simulink model "ExtDem_SelectParameter"  (R2016b)
settings: configuration reference "CodeGenConfigSet" (kept outside this file)
values from neighbouring files (symbols this model uses):
  ExtDem_facFdbk_CUR = Calibration.Parameter    [init_ExtDem_SelectParameter.m]
  ExtDem_facFdbk_CURX = Calibration.Parameter    [init_ExtDem_SelectParameter.m]
  ExtDem_facFdbkLimit_C = Calibration.Parameter    [init_ExtDem_SelectParameter.m]
  ExtDem_facFdbkParSet0_C = Calibration.Parameter    [init_ExtDem_SelectParameter.m]
  ExtDem_facFdbkParSet1_C = Calibration.Parameter    [init_ExtDem_SelectParameter.m]
  ExtDem_facFdbkParSet2_C = Calibration.Parameter    [init_ExtDem_SelectParameter.m]
  ExtDem_facFdbkParSet3_C = Calibration.Parameter    [init_ExtDem_SelectParameter.m]
  ExtDem_facFdbkParSet4_C = Calibration.Parameter    [init_ExtDem_SelectParameter.m]
  ExtDem_facFdbkParSet5_C = Calibration.Parameter    [init_ExtDem_SelectParameter.m]
  ExtDem_facFdbkParSet6_C = Calibration.Parameter    [init_ExtDem_SelectParameter.m]
  ExtDem_facFdbkParSet7_C = Calibration.Parameter    [init_ExtDem_SelectParameter.m]
  ExtDem_facNAvrgPT1CorFac_C = Calibration.Parameter    [init_ExtDem_SelectParameter.m]
  ExtDem_facTrqPT1CorFac_C = Calibration.Parameter    [init_ExtDem_SelectParameter.m]
  ExtDem_KiCorTempFac_MAP = Calibration.Parameter    [init_ExtDem_SelectParameter.m]
  ExtDem_KiCorTempFac_MAPX = Calibration.Parameter    [init_ExtDem_SelectParameter.m]
  ExtDem_KiCorTempFac_MAPY = Calibration.Parameter    [init_ExtDem_SelectParameter.m]
  ExtDem_KiCorTrqFac_MAP = Calibration.Parameter    [init_ExtDem_SelectParameter.m]
  ExtDem_KiCorTrqFac_MAPX = Calibration.Parameter    [init_ExtDem_SelectParameter.m]
  ExtDem_KiCorTrqFac_MAPY = Calibration.Parameter    [init_ExtDem_SelectParameter.m]
  ExtDem_KpCorTempFac_MAP = Calibration.Parameter    [init_ExtDem_SelectParameter.m]
  ExtDem_KpCorTempFac_MAPX = Calibration.Parameter    [init_ExtDem_SelectParameter.m]
  ExtDem_KpCorTempFac_MAPY = Calibration.Parameter    [init_ExtDem_SelectParameter.m]
  ExtDem_KpCorTrqFac_MAP = Calibration.Parameter    [init_ExtDem_SelectParameter.m]
  ExtDem_KpCorTrqFac_MAPX = Calibration.Parameter    [init_ExtDem_SelectParameter.m]
  ExtDem_KpCorTrqFac_MAPY = Calibration.Parameter    [init_ExtDem_SelectParameter.m]
  ExtDem_Par0Cfg_C = Calibration.Parameter    [init_ExtDem_SelectParameter.m]
  ExtDem_Par0dnAccLim_C = Calibration.Parameter    [init_ExtDem_SelectParameter.m]
  ExtDem_Par0dnDeclLim_C = Calibration.Parameter    [init_ExtDem_SelectParameter.m]
  ExtDem_Par0dnDeclLimBrk_C = Calibration.Parameter    [init_ExtDem_SelectParameter.m]
  ExtDem_Par0FacFdbkTrqLosHi_C = Calibration.Parameter    [init_ExtDem_SelectParameter.m]
  ExtDem_Par0FacFdbkTrqLosLo_C = Calibration.Parameter    [init_ExtDem_SelectParameter.m]
  ExtDem_Par0IKi_C = Calibration.Parameter    [init_ExtDem_SelectParameter.m]
  ExtDem_Par0IKiNeg_C = Calibration.Parameter    [init_ExtDem_SelectParameter.m]
  ExtDem_Par0IKiPos_C = Calibration.Parameter    [init_ExtDem_SelectParameter.m]
  ExtDem_Par0InrtVeh_C = Calibration.Parameter    [init_ExtDem_SelectParameter.m]
  ExtDem_Par0nIWinNeg_C = Calibration.Parameter    [init_ExtDem_SelectParameter.m]
  ExtDem_Par0nIWinPos_C = Calibration.Parameter    [init_ExtDem_SelectParameter.m]
  ExtDem_Par0nPWinNeg_C = Calibration.Parameter    [init_ExtDem_SelectParameter.m]
  ExtDem_Par0nPWinPos_C = Calibration.Parameter    [init_ExtDem_SelectParameter.m]
  ExtDem_Par0PKp_C = Calibration.Parameter    [init_ExtDem_SelectParameter.m]
  ExtDem_Par0PKpNeg_C = Calibration.Parameter    [init_ExtDem_SelectParameter.m]
  ExtDem_Par0PKpPos_C = Calibration.Parameter    [init_ExtDem_SelectParameter.m]
  ExtDem_Par0TiFltTrqLosEst_C = Calibration.Parameter    [init_ExtDem_SelectParameter.m]
  ExtDem_Par1Cfg_C = Calibration.Parameter    [init_ExtDem_SelectParameter.m]
  ExtDem_Par1dnAccLim_C = Calibration.Parameter    [init_ExtDem_SelectParameter.m]
  ExtDem_Par1dnDeclLim_C = Calibration.Parameter    [init_ExtDem_SelectParameter.m]
  ExtDem_Par1dnDeclLimBrk_C = Calibration.Parameter    [init_ExtDem_SelectParameter.m]
  ExtDem_Par1FacFdbkTrqLosHi_C = Calibration.Parameter    [init_ExtDem_SelectParameter.m]
  ExtDem_Par1FacFdbkTrqLosLo_C = Calibration.Parameter    [init_ExtDem_SelectParameter.m]
  ExtDem_Par1IKi_C = Calibration.Parameter    [init_ExtDem_SelectParameter.m]
  ExtDem_Par1IKiNeg_C = Calibration.Parameter    [init_ExtDem_SelectParameter.m]
  ExtDem_Par1IKiPos_C = Calibration.Parameter    [init_ExtDem_SelectParameter.m]
  ExtDem_Par1InrtVeh_C = Calibration.Parameter    [init_ExtDem_SelectParameter.m]
  ExtDem_Par1nIWinNeg_C = Calibration.Parameter    [init_ExtDem_SelectParameter.m]
  ExtDem_Par1nIWinPos_C = Calibration.Parameter    [init_ExtDem_SelectParameter.m]
  ExtDem_Par1nPWinNeg_C = Calibration.Parameter    [init_ExtDem_SelectParameter.m]
  ExtDem_Par1nPWinPos_C = Calibration.Parameter    [init_ExtDem_SelectParameter.m]
  ExtDem_Par1PKp_C = Calibration.Parameter    [init_ExtDem_SelectParameter.m]
  ExtDem_Par1PKpNeg_C = Calibration.Parameter    [init_ExtDem_SelectParameter.m]
  ExtDem_Par1PKpPos_C = Calibration.Parameter    [init_ExtDem_SelectParameter.m]
  ExtDem_Par1TiFltTrqLosEst_C = Calibration.Parameter    [init_ExtDem_SelectParameter.m]
  ExtDem_Par2Cfg_C = Calibration.Parameter    [init_ExtDem_SelectParameter.m]
  ExtDem_Par2dnAccLim_C = Calibration.Parameter    [init_ExtDem_SelectParameter.m]
  ExtDem_Par2dnDeclLim_C = Calibration.Parameter    [init_ExtDem_SelectParameter.m]
  ExtDem_Par2dnDeclLimBrk_C = Calibration.Parameter    [init_ExtDem_SelectParameter.m]
  ExtDem_Par2FacFdbkTrqLosHi_C = Calibration.Parameter    [init_ExtDem_SelectParameter.m]
  ExtDem_Par2FacFdbkTrqLosLo_C = Calibration.Parameter    [init_ExtDem_SelectParameter.m]
  ExtDem_Par2IKi_C = Calibration.Parameter    [init_ExtDem_SelectParameter.m]
  ExtDem_Par2IKiNeg_C = Calibration.Parameter    [init_ExtDem_SelectParameter.m]
  ExtDem_Par2IKiPos_C = Calibration.Parameter    [init_ExtDem_SelectParameter.m]
  ExtDem_Par2InrtVeh_C = Calibration.Parameter    [init_ExtDem_SelectParameter.m]
  ExtDem_Par2nIWinNeg_C = Calibration.Parameter    [init_ExtDem_SelectParameter.m]
  ExtDem_Par2nIWinPos_C = Calibration.Parameter    [init_ExtDem_SelectParameter.m]
  ExtDem_Par2nPWinNeg_C = Calibration.Parameter    [init_ExtDem_SelectParameter.m]
  ExtDem_Par2nPWinPos_C = Calibration.Parameter    [init_ExtDem_SelectParameter.m]
  ExtDem_Par2PKp_C = Calibration.Parameter    [init_ExtDem_SelectParameter.m]
  ExtDem_Par2PKpNeg_C = Calibration.Parameter    [init_ExtDem_SelectParameter.m]
  ExtDem_Par2PKpPos_C = Calibration.Parameter    [init_ExtDem_SelectParameter.m]
  ExtDem_Par2TiFltTrqLosEst_C = Calibration.Parameter    [init_ExtDem_SelectParameter.m]
  ExtDem_Par3Cfg_C = Calibration.Parameter    [init_ExtDem_SelectParameter.m]
  ExtDem_Par3dnAccLim_C = Calibration.Parameter    [init_ExtDem_SelectParameter.m]
  ExtDem_Par3dnDeclLim_C = Calibration.Parameter    [init_ExtDem_SelectParameter.m]
  ExtDem_Par3dnDeclLimBrk_C = Calibration.Parameter    [init_ExtDem_SelectParameter.m]
  ExtDem_Par3FacFdbkTrqLosHi_C = Calibration.Parameter    [init_ExtDem_SelectParameter.m]
  ExtDem_Par3FacFdbkTrqLosLo_C = Calibration.Parameter    [init_ExtDem_SelectParameter.m]
  ExtDem_Par3IKi_C = Calibration.Parameter    [init_ExtDem_SelectParameter.m]
  ExtDem_Par3IKiNeg_C = Calibration.Parameter    [init_ExtDem_SelectParameter.m]
  ExtDem_Par3IKiPos_C = Calibration.Parameter    [init_ExtDem_SelectParameter.m]
  ExtDem_Par3InrtVeh_C = Calibration.Parameter    [init_ExtDem_SelectParameter.m]
  ExtDem_Par3nIWinNeg_C = Calibration.Parameter    [init_ExtDem_SelectParameter.m]
  ExtDem_Par3nIWinPos_C = Calibration.Parameter    [init_ExtDem_SelectParameter.m]
  ExtDem_Par3nPWinNeg_C = Calibration.Parameter    [init_ExtDem_SelectParameter.m]
  ExtDem_Par3nPWinPos_C = Calibration.Parameter    [init_ExtDem_SelectParameter.m]
  ExtDem_Par3PKp_C = Calibration.Parameter    [init_ExtDem_SelectParameter.m]
  ExtDem_Par3PKpNeg_C = Calibration.Parameter    [init_ExtDem_SelectParameter.m]
  ExtDem_Par3PKpPos_C = Calibration.Parameter    [init_ExtDem_SelectParameter.m]
  ExtDem_Par3TiFltTrqLosEst_C = Calibration.Parameter    [init_ExtDem_SelectParameter.m]
  ExtDem_Par4Cfg_C = Calibration.Parameter    [init_ExtDem_SelectParameter.m]
  ExtDem_Par4dnAccLim_C = Calibration.Parameter    [init_ExtDem_SelectParameter.m]
  ExtDem_Par4dnDeclLim_C = Calibration.Parameter    [init_ExtDem_SelectParameter.m]
  ExtDem_Par4dnDeclLimBrk_C = Calibration.Parameter    [init_ExtDem_SelectParameter.m]
  ExtDem_Par4FacFdbkTrqLosHi_C = Calibration.Parameter    [init_ExtDem_SelectParameter.m]
  ExtDem_Par4FacFdbkTrqLosLo_C = Calibration.Parameter    [init_ExtDem_SelectParameter.m]
  ExtDem_Par4IKi_C = Calibration.Parameter    [init_ExtDem_SelectParameter.m]
  ExtDem_Par4IKiNeg_C = Calibration.Parameter    [init_ExtDem_SelectParameter.m]
  ExtDem_Par4IKiPos_C = Calibration.Parameter    [init_ExtDem_SelectParameter.m]
  ExtDem_Par4InrtVeh_C = Calibration.Parameter    [init_ExtDem_SelectParameter.m]
  ExtDem_Par4nIWinNeg_C = Calibration.Parameter    [init_ExtDem_SelectParameter.m]
  ExtDem_Par4nIWinPos_C = Calibration.Parameter    [init_ExtDem_SelectParameter.m]
  ExtDem_Par4nPWinNeg_C = Calibration.Parameter    [init_ExtDem_SelectParameter.m]
  ExtDem_Par4nPWinPos_C = Calibration.Parameter    [init_ExtDem_SelectParameter.m]
  ExtDem_Par4PKp_C = Calibration.Parameter    [init_ExtDem_SelectParameter.m]
  ExtDem_Par4PKpNeg_C = Calibration.Parameter    [init_ExtDem_SelectParameter.m]
  ExtDem_Par4PKpPos_C = Calibration.Parameter    [init_ExtDem_SelectParameter.m]
  ExtDem_Par4TiFltTrqLosEst_C = Calibration.Parameter    [init_ExtDem_SelectParameter.m]
  ExtDem_Par5Cfg_C = Calibration.Parameter    [init_ExtDem_SelectParameter.m]
  ExtDem_Par5dnAccLim_C = Calibration.Parameter    [init_ExtDem_SelectParameter.m]
  ExtDem_Par5dnDeclLim_C = Calibration.Parameter    [init_ExtDem_SelectParameter.m]
  ExtDem_Par5dnDeclLimBrk_C = Calibration.Parameter    [init_ExtDem_SelectParameter.m]
  ExtDem_Par5FacFdbkTrqLosHi_C = Calibration.Parameter    [init_ExtDem_SelectParameter.m]
  ... (+56 more)
libraries: CXLib x7
(part 1 of 2)
settings Model: Creator=dulinggang  LastModifiedBy=xuxingpei
settings ConfigSetRef: SourceLocation=Base Workspace

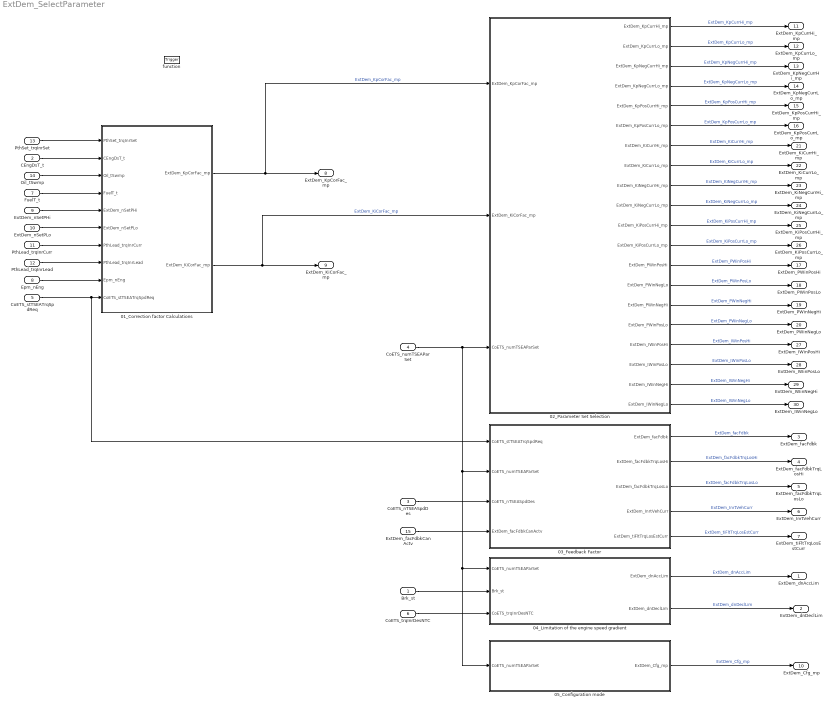
== system ExtDem_SelectParameter ==
  Brk_st : Inport  Description=Brake switch state  OutMin=0  OutMax=255  OutDataTypeStr=State_uint8
  CEngDsT_t : Inport  Tag=deg  Description=engine coolant temperature after filter  Port=2  OutMin=-200  OutMax=200  OutDataTypeStr=Temp_deg
  CoETS_nTSEASpdDes : Inport  Tag=rpm  Description=The desired/control engine speed requested from TSC1 CAN messages  Port=3  OutMin=0  OutMax=6000  OutDataTypeStr=EngSpeed_rpm
  CoETS_numTSEAParSet : Inport  Description=Number of requested parameter set for Engine speed governor  Port=4  OutMin=0  OutMax=255  OutDataTypeStr=State_uint8
  CoETS_stTSEATrqSpdReq : Inport  Description=Status of information about torque and speed intervention  Port=5  OutMin=0  OutMax=65535  OutDataTypeStr=State_uint16
  CoETS_trqInrDesNTC : Inport  Tag=Nm  Description=Additional desired engine friction Nm  Port=6  OutMin=-3276  OutMax=3276  OutDataTypeStr=Trq_Nm
  FuelT_t : Inport  Tag=deg  Description=EngPrt_PrtLimOvht:Temperature of fuel  Port=7  OutMin=-50  OutMax=150  OutDataTypeStr=Temp_deg
  Epm_nEng : Inport  Tag=rpm  Description=Engine speed  Port=8  OutMin=0  OutMax=6000  OutDataTypeStr=EngSpeed_rpm
  ExtDem_nSetPHi : Inport  Tag=rpm  Description=Higher limit of external demand set point speed  Port=9  OutMin=0  OutMax=6000  OutDataTypeStr=EngSpeed_rpm
  ExtDem_nSetPLo : Inport  Tag=rpm  Description=Lower limit of external demand set point speed  Port=10  OutMin=0  OutMax=6000  OutDataTypeStr=EngSpeed_rpm
  PthLead_trqInrCurr : Inport  Tag=Nm  Description=Actual percent engine torque  Port=11  OutMin=-3000  OutMax=3000  OutDataTypeStr=Trq_Nm
  PthLead_trqInrLead : Inport  Tag=Nm  Description=Inner torque lead value  Port=12  OutMin=-3000  OutMax=3000  OutDataTypeStr=Trq_Nm
  PthSet_trqInrSet : Inport  Tag=Nm  Description=Inner torque set value after monitoring limitation  Port=13  OutMin=-3000  OutMax=3276.7  OutDataTypeStr=Trq_Nm
  Oil_tSwmp : Inport  Tag=deg  Description=Oil temperature in oil sump  Port=14  OutMin=-50  OutMax=200  OutDataTypeStr=Temp_deg
  ExtDem_facFdbkCanActv : Inport  Tag=rpm/Nm  Description=External intervention feedback factor from CAN  Port=15  OutMin=-20  OutMax=20  OutDataTypeStr=FdbkNm2rpm_rpm_Nm
  function : TriggerPort  TriggerType=function-call  VariantControl=Variant
  "01_Correction factor Calculations " : Subsystem
  02_Parameter Set Selection : Subsystem
  "03_Feedback Factor " : Subsystem
  "04_Limitation of the engine speed gradient " : Subsystem
  "05_Conﬁguration mode " : Subsystem
  ExtDem_dnAccLim : Outport  Tag=rpm/s  Description=Maximum permissible acceleration (Engine speed)  OutMin=-12000  OutMax=12000  OutDataTypeStr=EngSpeed_rpm_s
  ExtDem_dnDeclLim : Outport  Tag=rpm/s  Description=Maximum permissible deceleration (Engine speed)  Port=2  OutMin=-12000  OutMax=12000  OutDataTypeStr=EngSpeed_rpm_s
  ExtDem_facFdbk : Outport  Tag=rpm/Nm  Description=External intervention feedback factor  Port=3  OutMin=-20  OutMax=20  OutDataTypeStr=FdbkNm2rpm_rpm_Nm
  ExtDem_facFdbkTrqLosHi : Outport  Tag=rpm/Nm  Description=inner feedback factor for the upper setpoint  Port=4  OutMin=-20  OutMax=20  OutDataTypeStr=FdbkNm2rpm_rpm_Nm
  ExtDem_facFdbkTrqLosLo : Outport  Tag=rpm/Nm  Description=inner feedback factor for the lower setpoint  Port=5  OutMin=-20  OutMax=20  OutDataTypeStr=FdbkNm2rpm_rpm_Nm
  ExtDem_InrtVehCurr : Outport  Tag=Nm/(rpm/s)  Description=Mass inirtia for EISGov torque loss estimation  Port=6  OutMin=-50  OutMax=50  OutDataTypeStr=HLSDem_Inrt
  ExtDem_tiFltTrqLosEstCurr : Outport  Tag=s  Description=Time constant for EISGov torque loss calculation  Port=7  OutMin=-180  OutMax=180  OutDataTypeStr=Time_s
  ExtDem_KpCorFac_mp : Outport  Description=Current small signal gain for the P component  Port=8  OutMin=-30  OutMax=30  OutDataTypeStr=Factor
  ExtDem_KiCorFac_mp : Outport  Description=Correction factor for I gain  Port=9  OutMin=-30  OutMax=30  OutDataTypeStr=Factor
  ExtDem_Cfg_mp : Outport  Description=Configuration for EISGov structure  Port=10  OutMin=0  OutMax=255  OutDataTypeStr=State_uint8
  ExtDem_KpCurrHi_mp : Outport  Tag=Nm/rpm  Description=Current small signal gain for the P higher component  Port=11  OutMin=-10000  OutMax=10000  OutDataTypeStr=HLSDem_Kp
  ExtDem_KpCurrLo_mp : Outport  Tag=Nm/rpm  Description=Current small signal gain for the P lower component  Port=12  OutMin=-10000  OutMax=10000  OutDataTypeStr=HLSDem_Kp
  ExtDem_KpNegCurrHi_mp : Outport  Tag=Nm/rpm  Description=Current negative large signal gain for the P higher component  Port=13  OutMin=-10000  OutMax=10000  OutDataTypeStr=HLSDem_Kp
  ExtDem_KpNegCurrLo_mp : Outport  Tag=Nm/rpm  Description=Current negative large signal gain for the lower P component  Port=14  OutMin=-10000  OutMax=10000  OutDataTypeStr=HLSDem_Kp
  ExtDem_KpPosCurrHi_mp : Outport  Tag=Nm/rpm  Description=Current positive large signal gain for the P higher component  Port=15  OutMin=-10000  OutMax=10000  OutDataTypeStr=HLSDem_Kp
  ExtDem_KpPosCurrLo_mp : Outport  Tag=Nm/rpm  Description=Current positive large signal gain for the P lower component  Port=16  OutMin=-10000  OutMax=10000  OutDataTypeStr=HLSDem_Kp
  ExtDem_PWinPosHi : Outport  Tag=rpm  Description=Positive small signal window for proportional higher component  Port=17  OutMin=-1000  OutMax=1000  OutDataTypeStr=EngSpeed_rpm
  ExtDem_PWinPosLo : Outport  Tag=rpm  Description=Positive small signal window for proportional lower component  Port=18  OutMin=-1000  OutMax=1000  OutDataTypeStr=EngSpeed_rpm
  ExtDem_PWinNegHi : Outport  Tag=rpm  Description=Negative small signal window for proportional higher component  Port=19  OutMin=-1000  OutMax=1000  OutDataTypeStr=EngSpeed_rpm
  ExtDem_PWinNegLo : Outport  Tag=rpm  Description=Negative small signal window for proportional lower component  Port=20  OutMin=-1000  OutMax=1000  OutDataTypeStr=EngSpeed_rpm
  ExtDem_KiCurrHi_mp : Outport  Tag=Nm/(rpm*s)  Description=Current small signal gain for the I higher component  Port=21  OutMin=-18000  OutMax=18000  OutDataTypeStr=HLSDem_Ki
  ExtDem_KiCurrLo_mp : Outport  Tag=Nm/(rpm*s)  Description=Current small signal gain for the I lower component  Port=22  OutMin=-18000  OutMax=18000  OutDataTypeStr=HLSDem_Ki
  ExtDem_KiNegCurrHi_mp : Outport  Tag=Nm/(rpm*s)  Description=Current negative large signal gain for the I higher component  Port=23  OutMin=-18000  OutMax=18000  OutDataTypeStr=HLSDem_Ki
  ExtDem_KiNegCurrLo_mp : Outport  Tag=Nm/(rpm*s)  Description=Current negative large signal gain for the I lower component  Port=24  OutMin=-18000  OutMax=18000  OutDataTypeStr=HLSDem_Ki
  ExtDem_KiPosCurrHi_mp : Outport  Tag=Nm/(rpm*s)  Description=Current positive large signal gain for the I higher component  Port=25  OutMin=-18000  OutMax=18000  OutDataTypeStr=HLSDem_Ki
  ExtDem_KiPosCurrLo_mp : Outport  Tag=Nm/(rpm*s)  Description=Current positive large signal gain for the I lower component  Port=26  OutMin=-18000  OutMax=18000  OutDataTypeStr=HLSDem_Ki
  ExtDem_IWinPosHi : Outport  Tag=rpm  Description=Positive small signal window for integral higher component  Port=27  OutMin=-1000  OutMax=1000  OutDataTypeStr=EngSpeed_rpm
  ExtDem_IWinPosLo : Outport  Tag=rpm  Description=Positive small signal window for integral lower component  Port=28  OutMin=-1000  OutMax=1000  OutDataTypeStr=EngSpeed_rpm
  ExtDem_IWinNegHi : Outport  Tag=rpm  Description=Negative small signal window for integral higher component  Port=29  OutMin=-1000  OutMax=1000  OutDataTypeStr=EngSpeed_rpm
  ExtDem_IWinNegLo : Outport  Tag=rpm  Description=Negative small signal window for integral lower component  Port=30  OutMin=-1000  OutMax=1000  OutDataTypeStr=EngSpeed_rpm
  wires:
  "03_Feedback Factor "/1(ExtDem_facFdbk) -> ExtDem_facFdbk/1  "ExtDem_facFdbk"
  "03_Feedback Factor "/2(ExtDem_facFdbkTrqLosHi) -> ExtDem_facFdbkTrqLosHi/1  "ExtDem_facFdbkTrqLosHi"
  "03_Feedback Factor "/3(ExtDem_facFdbkTrqLosLo) -> ExtDem_facFdbkTrqLosLo/1  "ExtDem_facFdbkTrqLosLo"
  "03_Feedback Factor "/4(ExtDem_InrtVehCurr) -> ExtDem_InrtVehCurr/1  "ExtDem_InrtVehCurr"
  "01_Correction factor Calculations "/1(ExtDem_KpCorFac_mp) -> ExtDem_KpCorFac_mp/1, 02_Parameter Set Selection/1(ExtDem_KpCorFac_mp)  "ExtDem_KpCorFac_mp"
  "01_Correction factor Calculations "/2(ExtDem_KiCorFac_mp) -> ExtDem_KiCorFac_mp/1, 02_Parameter Set Selection/2(ExtDem_KiCorFac_mp)  "ExtDem_KiCorFac_mp"
  "05_Conﬁguration mode "/1(ExtDem_Cfg_mp) -> ExtDem_Cfg_mp/1  "ExtDem_Cfg_mp"
  CoETS_stTSEATrqSpdReq/1 -> "03_Feedback Factor "/1(CoETS_stTSEATrqSpdReq), "01_Correction factor Calculations "/10(CoETS_stTSEATrqSpdReq)
  ExtDem_nSetPHi/1 -> "01_Correction factor Calculations "/5(ExtDem_nSetPHi)
  PthLead_trqInrCurr/1 -> "01_Correction factor Calculations "/7(PthLead_trqInrCurr)
  PthLead_trqInrLead/1 -> "01_Correction factor Calculations "/8(PthLead_trqInrLead)
  PthSet_trqInrSet/1 -> "01_Correction factor Calculations "/1(PthSet_trqInrSet)
  CEngDsT_t/1 -> "01_Correction factor Calculations "/2(CEngDsT_t)
  Oil_tSwmp/1 -> "01_Correction factor Calculations "/3(Oil_tSwmp)
  FuelT_t/1 -> "01_Correction factor Calculations "/4(FuelT_t)
  CoETS_numTSEAParSet/1 -> "03_Feedback Factor "/2(CoETS_numTSEAParSet), "05_Conﬁguration mode "/1(CoETS_numTSEAParSet), "04_Limitation of the engine speed gradient "/1(CoETS_numTSEAParSet), 02_Parameter Set Selection/3(CoETS_numTSEAParSet)
  CoETS_nTSEASpdDes/1 -> "03_Feedback Factor "/3(CoETS_nTSEASpdDes)
  Brk_st/1 -> "04_Limitation of the engine speed gradient "/2(Brk_st)
  CoETS_trqInrDesNTC/1 -> "04_Limitation of the engine speed gradient "/3(CoETS_trqInrDesNTC)
  "04_Limitation of the engine speed gradient "/1(ExtDem_dnAccLim) -> ExtDem_dnAccLim/1  "ExtDem_dnAccLim"
  "04_Limitation of the engine speed gradient "/2(ExtDem_dnDeclLim) -> ExtDem_dnDeclLim/1  "ExtDem_dnDeclLim"
  Epm_nEng/1 -> "01_Correction factor Calculations "/9(Epm_nEng)
  ExtDem_nSetPLo/1 -> "01_Correction factor Calculations "/6(ExtDem_nSetPLo)
  02_Parameter Set Selection/1(ExtDem_KpCurrHi_mp) -> ExtDem_KpCurrHi_mp/1  "ExtDem_KpCurrHi_mp"
  02_Parameter Set Selection/2(ExtDem_KpCurrLo_mp) -> ExtDem_KpCurrLo_mp/1  "ExtDem_KpCurrLo_mp"
  02_Parameter Set Selection/3(ExtDem_KpNegCurrHi_mp) -> ExtDem_KpNegCurrHi_mp/1  "ExtDem_KpNegCurrHi_mp"
  02_Parameter Set Selection/4(ExtDem_KpNegCurrLo_mp) -> ExtDem_KpNegCurrLo_mp/1  "ExtDem_KpNegCurrLo_mp"
  02_Parameter Set Selection/5(ExtDem_KpPosCurrHi_mp) -> ExtDem_KpPosCurrHi_mp/1  "ExtDem_KpPosCurrHi_mp"
  02_Parameter Set Selection/6(ExtDem_KpPosCurrLo_mp) -> ExtDem_KpPosCurrLo_mp/1  "ExtDem_KpPosCurrLo_mp"
  02_Parameter Set Selection/7(ExtDem_KiCurrHi_mp) -> ExtDem_KiCurrHi_mp/1  "ExtDem_KiCurrHi_mp"
  02_Parameter Set Selection/8(ExtDem_KiCurrLo_mp) -> ExtDem_KiCurrLo_mp/1  "ExtDem_KiCurrLo_mp"
  02_Parameter Set Selection/9(ExtDem_KiNegCurrHi_mp) -> ExtDem_KiNegCurrHi_mp/1  "ExtDem_KiNegCurrHi_mp"
  02_Parameter Set Selection/10(ExtDem_KiNegCurrLo_mp) -> ExtDem_KiNegCurrLo_mp/1  "ExtDem_KiNegCurrLo_mp"
  02_Parameter Set Selection/11(ExtDem_KiPosCurrHi_mp) -> ExtDem_KiPosCurrHi_mp/1  "ExtDem_KiPosCurrHi_mp"
  02_Parameter Set Selection/12(ExtDem_KiPosCurrLo_mp) -> ExtDem_KiPosCurrLo_mp/1  "ExtDem_KiPosCurrLo_mp"
  ExtDem_facFdbkCanActv/1 -> "03_Feedback Factor "/4(ExtDem_facFdbkCanActv)
  "03_Feedback Factor "/5(ExtDem_tiFltTrqLosEstCurr) -> ExtDem_tiFltTrqLosEstCurr/1  "ExtDem_tiFltTrqLosEstCurr"
  02_Parameter Set Selection/17(ExtDem_IWinPosHi) -> ExtDem_IWinPosHi/1  "ExtDem_IWinPosHi"
  02_Parameter Set Selection/18(ExtDem_IWinPosLo) -> ExtDem_IWinPosLo/1  "ExtDem_IWinPosLo"
  02_Parameter Set Selection/19(ExtDem_IWinNegHi) -> ExtDem_IWinNegHi/1  "ExtDem_IWinNegHi"
  02_Parameter Set Selection/20(ExtDem_IWinNegLo) -> ExtDem_IWinNegLo/1  "ExtDem_IWinNegLo"
  02_Parameter Set Selection/13(ExtDem_PWinPosHi) -> ExtDem_PWinPosHi/1  "ExtDem_PWinPosHi"
  02_Parameter Set Selection/15(ExtDem_PWinNegHi) -> ExtDem_PWinNegHi/1  "ExtDem_PWinNegHi"
  02_Parameter Set Selection/14(ExtDem_PWinNegLo) -> ExtDem_PWinPosLo/1  "ExtDem_PWinPosLo"
  02_Parameter Set Selection/16(ExtDem_PWinPosLo) -> ExtDem_PWinNegLo/1  "ExtDem_PWinNegLo"

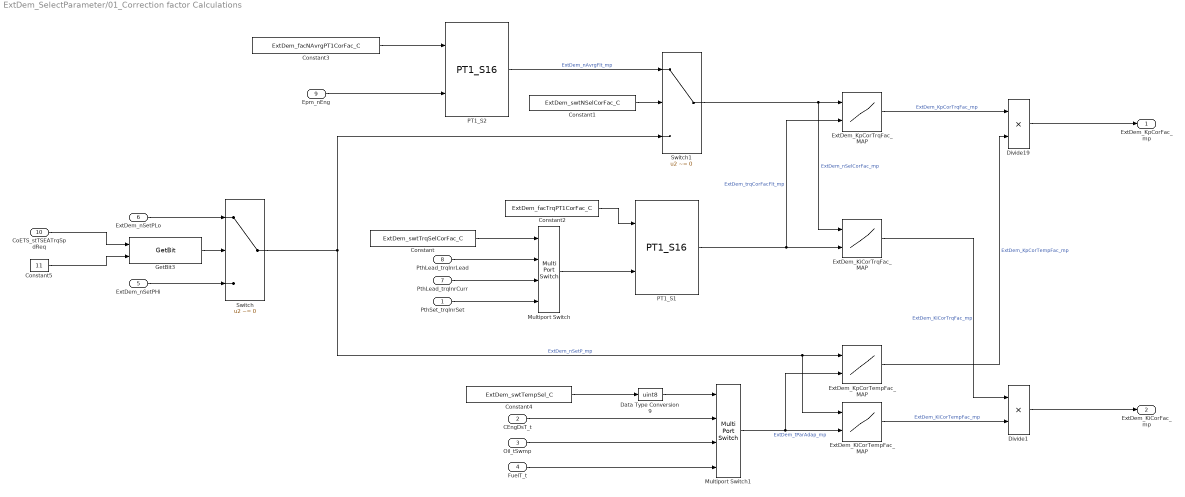
== system ExtDem_SelectParameter/01_Correction factor Calculations  ==
  PthSet_trqInrSet : Inport  Tag=Nm  Description=Inner torque set value after monitoring limitation  OutMin=-3000  OutMax=3276.7  OutDataTypeStr=Trq_Nm
  CEngDsT_t : Inport  Tag=deg  Description=engine coolant temperature after filter  Port=2  OutMin=-200  OutMax=200  OutDataTypeStr=Temp_deg
  Oil_tSwmp : Inport  Tag=deg  Description=Oil temperature in oil sump  Port=3  OutMin=-50  OutMax=200  OutDataTypeStr=Temp_deg
  FuelT_t : Inport  Tag=deg  Description=Engine temperature field  Port=4  OutMin=-3000  OutMax=3000  OutDataTypeStr=Temp_deg
  ExtDem_nSetPHi : Inport  Tag=rpm  Description=Higher limit of external demand set point speed  Port=5  OutMin=0  OutMax=6000  OutDataTypeStr=EngSpeed_rpm
  ExtDem_nSetPLo : Inport  Tag=rpm  Description=Lower limit of external demand set point speed  Port=6  OutMin=0  OutMax=6000  OutDataTypeStr=EngSpeed_rpm
  PthLead_trqInrCurr : Inport  Tag=Nm  Description=Actual percent engine torque  Port=7  OutMin=-3000  OutMax=3000  OutDataTypeStr=Trq_Nm
  PthLead_trqInrLead : Inport  Tag=Nm  Description=Inner torque lead value  Port=8  OutMin=-3000  OutMax=3000  OutDataTypeStr=Trq_Nm
  Epm_nEng : Inport  Tag=rpm  Description=Engine speed  Port=9  OutMin=0  OutMax=6000  OutDataTypeStr=EngSpeed_rpm
  CoETS_stTSEATrqSpdReq : Inport  Description=Status of information about torque and speed intervention  Port=10  OutMin=0  OutMax=65535  OutDataTypeStr=State_uint16
  Constant : Constant  Value=ExtDem_swtTrqSelCorFac_C
  Constant1 : Constant  Value=ExtDem_swtNSelCorFac_C
  Constant2 : Constant  Value=ExtDem_facTrqPT1CorFac_C
  Constant3 : Constant  Value=ExtDem_facNAvrgPT1CorFac_C
  Constant4 : Constant  Value=ExtDem_swtTempSel_C
  Constant5 : Constant  Value=11  OutDataTypeStr=Inherit: Inherit via back propagation
  Data Type Conversion9 : DataTypeConversion  OutDataTypeStr=uint8
  Divide1 : Product  Inputs=**  OutDataTypeStr=Factor  SaturateOnIntegerOverflow=on
  Divide19 : Product  Inputs=**  OutDataTypeStr=Factor  SaturateOnIntegerOverflow=on
  ExtDem_KiCorTempFac_MAP : Lookup_n-D  BreakpointsForDimension1=ExtDem_KiCorTempFac_MAPX  BreakpointsForDimension2=ExtDem_KiCorTempFac_MAPY  BeginIndexSearchUsingPreviousIndexResult=on  Table=ExtDem_KiCorTempFac_MAP  ExtrapMethod=Clip  UseLastTableValue=on  InternalRulePriority=Speed  OutDataTypeStr=Inherit: Inherit via back propagation  RndMeth=Simplest  SaturateOnIntegerOverflow=on
  ExtDem_KiCorTrqFac_MAP : Lookup_n-D  BreakpointsForDimension1=ExtDem_KiCorTrqFac_MAPX  BreakpointsForDimension2=ExtDem_KiCorTrqFac_MAPY  BeginIndexSearchUsingPreviousIndexResult=on  Table=ExtDem_KiCorTrqFac_MAP  ExtrapMethod=Clip  UseLastTableValue=on  InternalRulePriority=Speed  OutDataTypeStr=Inherit: Inherit via back propagation  RndMeth=Simplest  SaturateOnIntegerOverflow=on
  ExtDem_KpCorTempFac_MAP : Lookup_n-D  BreakpointsForDimension1=ExtDem_KpCorTempFac_MAPX  BreakpointsForDimension2=ExtDem_KpCorTempFac_MAPY  BeginIndexSearchUsingPreviousIndexResult=on  Table=ExtDem_KpCorTempFac_MAP  ExtrapMethod=Clip  UseLastTableValue=on  InternalRulePriority=Speed  OutDataTypeStr=Inherit: Inherit via back propagation  RndMeth=Simplest  SaturateOnIntegerOverflow=on
  ExtDem_KpCorTrqFac_MAP : Lookup_n-D  BreakpointsForDimension1=ExtDem_KpCorTrqFac_MAPX  BreakpointsForDimension2=ExtDem_KpCorTrqFac_MAPY  BeginIndexSearchUsingPreviousIndexResult=on  Table=ExtDem_KpCorTrqFac_MAP  ExtrapMethod=Clip  UseLastTableValue=on  InternalRulePriority=Speed  OutDataTypeStr=Inherit: Inherit via back propagation  RndMeth=Simplest  SaturateOnIntegerOverflow=on
  GetBit3 : CXLib/GetBit  dataTypeString=uint16  dataLength=0
      settings: AttributesFormatString=Get bit from %<dataTypeString>
  Multiport Switch : MultiPortSwitch  DataPortOrder=Zero-based contiguous
  Multiport Switch1 : MultiPortSwitch  DataPortOrder=Zero-based contiguous
  PT1_S1 : CXLib/PT1_S16
  PT1_S2 : CXLib/PT1_S16
  Switch : Switch  Criteria=u2 ~= 0
  Switch1 : Switch  Criteria=u2 ~= 0
  ExtDem_KpCorFac_mp : Outport  Description=Current small signal gain for the P component  OutMin=-30  OutMax=30  OutDataTypeStr=Factor
  ExtDem_KiCorFac_mp : Outport  Description=Correction factor for I gain  Port=2  OutMin=-30  OutMax=30  OutDataTypeStr=Factor
  wires:
  ExtDem_nSetPLo/1 -> Switch/1
  ExtDem_nSetPHi/1 -> Switch/3
  GetBit3/1 -> Switch/2
  Switch/1 -> Switch1/3, ExtDem_KiCorTempFac_MAP/1, ExtDem_KpCorTempFac_MAP/1  "ExtDem_nSetP_mp"
  PthSet_trqInrSet/1 -> Multiport Switch/4
  PthLead_trqInrCurr/1 -> Multiport Switch/3
  PthLead_trqInrLead/1 -> Multiport Switch/2
  Constant/1 -> Multiport Switch/1
  Multiport Switch/1 -> PT1_S1/2
  Epm_nEng/1 -> PT1_S2/2
  PT1_S2/1 -> Switch1/1  "ExtDem_nAvrgFlt_mp"
  Switch1/1 -> ExtDem_KiCorTrqFac_MAP/1, ExtDem_KpCorTrqFac_MAP/1  "ExtDem_nSelCorFac_mp"
  Constant1/1 -> Switch1/2
  Constant2/1 -> PT1_S1/1
  Constant3/1 -> PT1_S2/1
  ExtDem_KpCorTrqFac_MAP/1 -> Divide19/1  "ExtDem_KpCorTrqFac_mp"
  ExtDem_KiCorTrqFac_MAP/1 -> Divide1/1  "ExtDem_KiCorTrqFac_mp"
  CEngDsT_t/1 -> Multiport Switch1/2
  Oil_tSwmp/1 -> Multiport Switch1/3
  FuelT_t/1 -> Multiport Switch1/4
  Data Type Conversion9/1 -> Multiport Switch1/1
  Constant4/1 -> Data Type Conversion9/1
  Multiport Switch1/1 -> ExtDem_KiCorTempFac_MAP/2, ExtDem_KpCorTempFac_MAP/2  "ExtDem_tParAdap_mp"
  ExtDem_KpCorTempFac_MAP/1 -> Divide19/2  "ExtDem_KpCorTempFac_mp"
  ExtDem_KiCorTempFac_MAP/1 -> Divide1/2  "ExtDem_KiCorTempFac_mp"
  Divide19/1 -> ExtDem_KpCorFac_mp/1
  Divide1/1 -> ExtDem_KiCorFac_mp/1
  PT1_S1/1 -> ExtDem_KpCorTrqFac_MAP/2, ExtDem_KiCorTrqFac_MAP/2  "ExtDem_trqCorFacFlt_mp"
  Constant5/1 -> GetBit3/2
  CoETS_stTSEATrqSpdReq/1 -> GetBit3/1

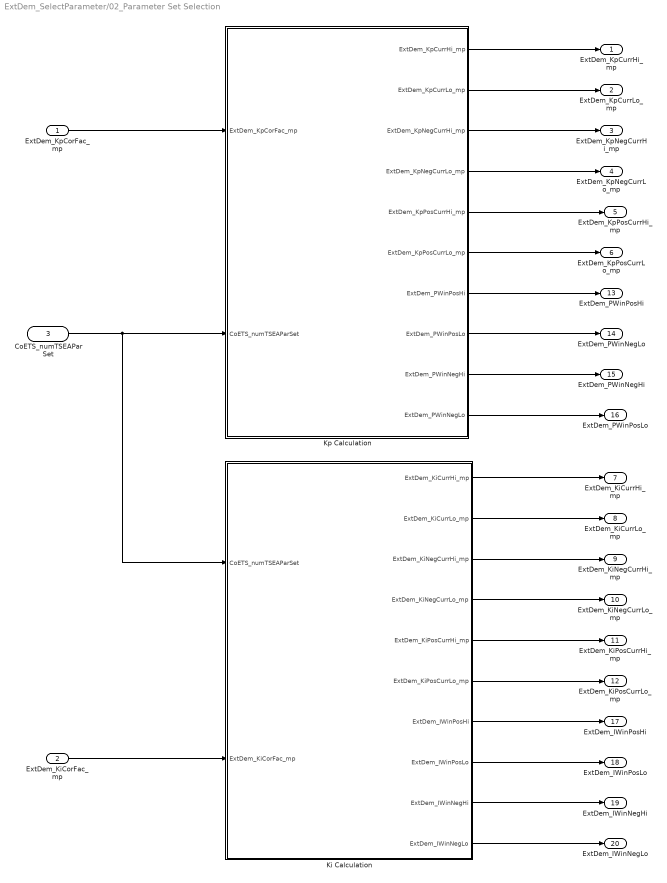
== system ExtDem_SelectParameter/02_Parameter Set Selection ==
  ExtDem_KpCorFac_mp : Inport  Description=Number of requested parameter set for Engine speed governor  OutMin=-30  OutMax=30  OutDataTypeStr=Factor
  ExtDem_KiCorFac_mp : Inport  Description=Number of requested parameter set for Engine speed governor  Port=2  OutMin=-30  OutMax=30  OutDataTypeStr=Factor
  CoETS_numTSEAParSet : Inport  Description=Number of requested parameter set for Engine speed governor  Port=3  OutMin=0  OutMax=255  OutDataTypeStr=uint8
  Ki Calculation : Subsystem
  "Kp Calculation " : Subsystem
  ExtDem_KpCurrHi_mp : Outport  Tag=Nm/rpm  Description=Current small signal gain for the P higher component  OutMin=-10000  OutMax=10000  OutDataTypeStr=HLSDem_Kp
  ExtDem_KpCurrLo_mp : Outport  Tag=Nm/rpm  Description=Current small signal gain for the P lower component  Port=2  OutMin=-10000  OutMax=10000  OutDataTypeStr=HLSDem_Kp
  ExtDem_KpNegCurrHi_mp : Outport  Tag=Nm/rpm  Description=Current negative large signal gain for the P higher component  Port=3  OutMin=-10000  OutMax=10000  OutDataTypeStr=HLSDem_Kp
  ExtDem_KpNegCurrLo_mp : Outport  Tag=Nm/rpm  Description=Current negative large signal gain for the lower P component  Port=4  OutMin=-10000  OutMax=10000  OutDataTypeStr=HLSDem_Kp
  ExtDem_KpPosCurrHi_mp : Outport  Tag=Nm/rpm  Description=Current positive large signal gain for the P higher component  Port=5  OutMin=-10000  OutMax=10000  OutDataTypeStr=HLSDem_Kp
  ExtDem_KpPosCurrLo_mp : Outport  Tag=Nm/rpm  Description=Current positive large signal gain for the P lower component  Port=6  OutMin=-10000  OutMax=10000  OutDataTypeStr=HLSDem_Kp
  ExtDem_KiCurrHi_mp : Outport  Tag=Nm/(rpm*s)  Description=Current small signal gain for the I higher component  Port=7  OutMin=-18000  OutMax=18000  OutDataTypeStr=HLSDem_Ki
  ExtDem_KiCurrLo_mp : Outport  Tag=Nm/(rpm*s)  Description=Current small signal gain for the I lower component  Port=8  OutMin=-18000  OutMax=18000  OutDataTypeStr=HLSDem_Ki
  ExtDem_KiNegCurrHi_mp : Outport  Tag=Nm/(rpm*s)  Description=Current negative large signal gain for the I higher component  Port=9  OutMin=-18000  OutMax=18000  OutDataTypeStr=HLSDem_Ki
  ExtDem_KiNegCurrLo_mp : Outport  Tag=Nm/(rpm*s)  Description=Current negative large signal gain for the I lower component  Port=10  OutMin=-18000  OutMax=18000  OutDataTypeStr=HLSDem_Ki
  ExtDem_KiPosCurrHi_mp : Outport  Tag=Nm/(rpm*s)  Description=Current positive large signal gain for the I higher component  Port=11  OutMin=-18000  OutMax=18000  OutDataTypeStr=HLSDem_Ki
  ExtDem_KiPosCurrLo_mp : Outport  Tag=Nm/(rpm*s)  Description=Current positive large signal gain for the I lower component  Port=12  OutMin=-18000  OutMax=18000  OutDataTypeStr=HLSDem_Ki
  ExtDem_PWinPosHi : Outport  Tag=rpm  Description=Positive small signal window for proportional higher component  Port=13  OutMin=-1000  OutMax=1000  OutDataTypeStr=EngSpeed_rpm
  ExtDem_PWinNegLo : Outport  Tag=rpm  Description=Negative small signal window for proportional lower component  Port=14  OutMin=-1000  OutMax=1000  OutDataTypeStr=EngSpeed_rpm
  ExtDem_PWinNegHi : Outport  Tag=rpm  Description=Negative small signal window for proportional higher component  Port=15  OutMin=-1000  OutMax=1000  OutDataTypeStr=EngSpeed_rpm
  ExtDem_PWinPosLo : Outport  Tag=rpm  Description=Positive small signal window for proportional lower component  Port=16  OutMin=-1000  OutMax=1000  OutDataTypeStr=EngSpeed_rpm
  ExtDem_IWinPosHi : Outport  Tag=rpm  Description=Positive small signal window for integral higher component  Port=17  OutMin=-1000  OutMax=1000  OutDataTypeStr=EngSpeed_rpm
  ExtDem_IWinPosLo : Outport  Tag=rpm  Description=Positive small signal window for integral lower component  Port=18  OutMin=-1000  OutMax=1000  OutDataTypeStr=EngSpeed_rpm
  ExtDem_IWinNegHi : Outport  Tag=rpm  Description=Negative small signal window for integral higher component  Port=19  OutMin=-1000  OutMax=1000  OutDataTypeStr=EngSpeed_rpm
  ExtDem_IWinNegLo : Outport  Tag=rpm  Description=Negative small signal window for integral lower component  Port=20  OutMin=-1000  OutMax=1000  OutDataTypeStr=EngSpeed_rpm
  wires:
  CoETS_numTSEAParSet/1 -> Ki Calculation/1(CoETS_numTSEAParSet), "Kp Calculation "/2(CoETS_numTSEAParSet)
  "Kp Calculation "/1(ExtDem_KpCurrHi_mp) -> ExtDem_KpCurrHi_mp/1
  "Kp Calculation "/2(ExtDem_KpCurrLo_mp) -> ExtDem_KpCurrLo_mp/1
  "Kp Calculation "/3(ExtDem_KpNegCurrHi_mp) -> ExtDem_KpNegCurrHi_mp/1
  "Kp Calculation "/4(ExtDem_KpNegCurrLo_mp) -> ExtDem_KpNegCurrLo_mp/1
  "Kp Calculation "/5(ExtDem_KpPosCurrHi_mp) -> ExtDem_KpPosCurrHi_mp/1
  "Kp Calculation "/6(ExtDem_KpPosCurrLo_mp) -> ExtDem_KpPosCurrLo_mp/1
  Ki Calculation/1(ExtDem_KiCurrHi_mp) -> ExtDem_KiCurrHi_mp/1
  Ki Calculation/2(ExtDem_KiCurrLo_mp) -> ExtDem_KiCurrLo_mp/1
  Ki Calculation/3(ExtDem_KiNegCurrHi_mp) -> ExtDem_KiNegCurrHi_mp/1
  Ki Calculation/4(ExtDem_KiNegCurrLo_mp) -> ExtDem_KiNegCurrLo_mp/1
  Ki Calculation/5(ExtDem_KiPosCurrHi_mp) -> ExtDem_KiPosCurrHi_mp/1
  Ki Calculation/6(ExtDem_KiPosCurrLo_mp) -> ExtDem_KiPosCurrLo_mp/1
  ExtDem_KpCorFac_mp/1 -> "Kp Calculation "/1(ExtDem_KpCorFac_mp)
  ExtDem_KiCorFac_mp/1 -> Ki Calculation/2(ExtDem_KiCorFac_mp)
  "Kp Calculation "/7(ExtDem_PWinPosHi) -> ExtDem_PWinPosHi/1
  "Kp Calculation "/9(ExtDem_PWinNegHi) -> ExtDem_PWinNegHi/1
  Ki Calculation/7(ExtDem_IWinPosHi) -> ExtDem_IWinPosHi/1
  Ki Calculation/8(ExtDem_IWinPosLo) -> ExtDem_IWinPosLo/1
  Ki Calculation/9(ExtDem_IWinNegHi) -> ExtDem_IWinNegHi/1
  Ki Calculation/10(ExtDem_IWinNegLo) -> ExtDem_IWinNegLo/1
  "Kp Calculation "/10(ExtDem_PWinNegLo) -> ExtDem_PWinPosLo/1
  "Kp Calculation "/8(ExtDem_PWinPosLo) -> ExtDem_PWinNegLo/1

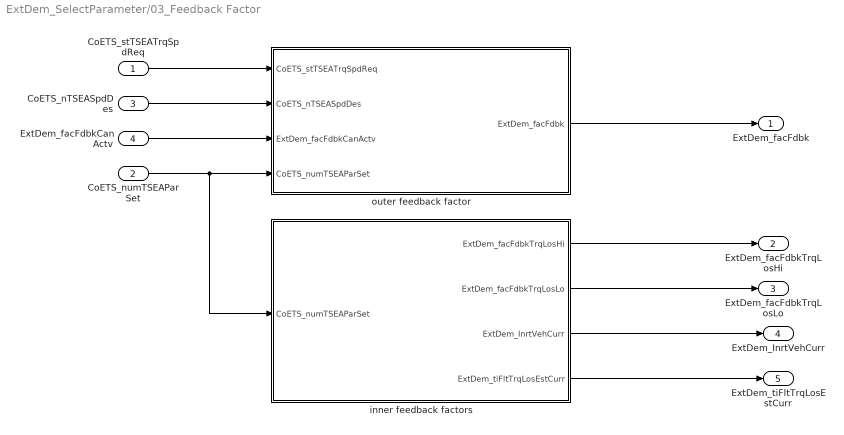
== system ExtDem_SelectParameter/03_Feedback Factor  ==
  CoETS_stTSEATrqSpdReq : Inport  Description=Status of information about torque and speed intervention  OutMin=0  OutMax=65535  OutDataTypeStr=State_uint16
  CoETS_numTSEAParSet : Inport  Description=Number of requested parameter set for Engine speed governor  Port=2  OutMin=0  OutMax=255  OutDataTypeStr=State_uint8
  CoETS_nTSEASpdDes : Inport  Tag=rpm  Description=The desired/control engine speed requested from TSC1 CAN messages  Port=3  OutMin=0  OutMax=6000  OutDataTypeStr=EngSpeed_rpm
  ExtDem_facFdbkCanActv : Inport  Tag=rpm/Nm  Description=External intervention feedback factor from CAN  Port=4  OutMin=-20  OutMax=20  OutDataTypeStr=FdbkNm2rpm_rpm_Nm
  " inner feedback factors " : Subsystem
  "outer feedback factor " : Subsystem
  ExtDem_facFdbk : Outport  Tag=rpm/Nm  Description=External intervention feedback factor  OutMin=-20  OutMax=20  OutDataTypeStr=FdbkNm2rpm_rpm_Nm
  ExtDem_facFdbkTrqLosHi : Outport  Tag=rpm/Nm  Description=inner feedback factor for the upper setpoint  Port=2  OutMin=-20  OutMax=20  OutDataTypeStr=FdbkNm2rpm_rpm_Nm
  ExtDem_facFdbkTrqLosLo : Outport  Tag=rpm/Nm  Description=inner feedback factor for the lower setpoint  Port=3  OutMin=-20  OutMax=20  OutDataTypeStr=FdbkNm2rpm_rpm_Nm
  ExtDem_InrtVehCurr : Outport  Tag=Nm/(rpm/s)  Description=Mass inirtia for EISGov torque loss estimation  Port=4  OutMin=-50  OutMax=50  OutDataTypeStr=HLSDem_Inrt
  ExtDem_tiFltTrqLosEstCurr : Outport  Tag=s  Description=Time constant for EISGov torque loss calculation  Port=5  OutMin=-180  OutMax=180  OutDataTypeStr=Time_s
  wires:
  CoETS_stTSEATrqSpdReq/1 -> "outer feedback factor "/1(CoETS_stTSEATrqSpdReq)
  CoETS_nTSEASpdDes/1 -> "outer feedback factor "/2(CoETS_nTSEASpdDes)
  "outer feedback factor "/1(ExtDem_facFdbk) -> ExtDem_facFdbk/1
  " inner feedback factors "/1(ExtDem_facFdbkTrqLosHi) -> ExtDem_facFdbkTrqLosHi/1
  " inner feedback factors "/2(ExtDem_facFdbkTrqLosLo) -> ExtDem_facFdbkTrqLosLo/1
  CoETS_numTSEAParSet/1 -> " inner feedback factors "/1(CoETS_numTSEAParSet), "outer feedback factor "/4(CoETS_numTSEAParSet)
  " inner feedback factors "/3(ExtDem_InrtVehCurr) -> ExtDem_InrtVehCurr/1
  ExtDem_facFdbkCanActv/1 -> "outer feedback factor "/3(ExtDem_facFdbkCanActv)
  " inner feedback factors "/4(ExtDem_tiFltTrqLosEstCurr) -> ExtDem_tiFltTrqLosEstCurr/1

== system ExtDem_SelectParameter/04_Limitation of the engine speed gradient  ==
  CoETS_numTSEAParSet : Inport  Description=Number of requested parameter set for Engine speed governor  OutMin=0  OutMax=255  OutDataTypeStr=State_uint8
  Brk_st : Inport  Description=Brake switch state  Port=2  OutMin=0  OutMax=255  OutDataTypeStr=State_uint8
  CoETS_trqInrDesNTC : Inport  Tag=Nm  Description=Additional desired engine friction Nm  Port=3  OutMin=-3276  OutMax=3276  OutDataTypeStr=Trq_Nm
  dnAccLim : Subsystem
  dnDecLim : Subsystem
  ExtDem_dnAccLim : Outport  Tag=rpm/s  Description=Maximum permissible acceleration (Engine speed)  OutMin=-12000  OutMax=12000  OutDataTypeStr=EngSpeed_rpm_s
  ExtDem_dnDeclLim : Outport  Tag=rpm/s  Description=Maximum permissible deceleration (Engine speed)  Port=2  OutMin=-12000  OutMax=12000  OutDataTypeStr=EngSpeed_rpm_s
  wires:
  CoETS_numTSEAParSet/1 -> dnDecLim/1(CoETS_numTSEAParSet), dnAccLim/1(CoETS_numTSEAParSet)
  dnAccLim/1(ExtDem_dnAccLim) -> ExtDem_dnAccLim/1
  dnDecLim/1(ExtDem_dnDeclLim) -> ExtDem_dnDeclLim/1
  Brk_st/1 -> dnDecLim/2(Brk_st)
  CoETS_trqInrDesNTC/1 -> dnDecLim/3(CoETS_trqInrDesNTC)

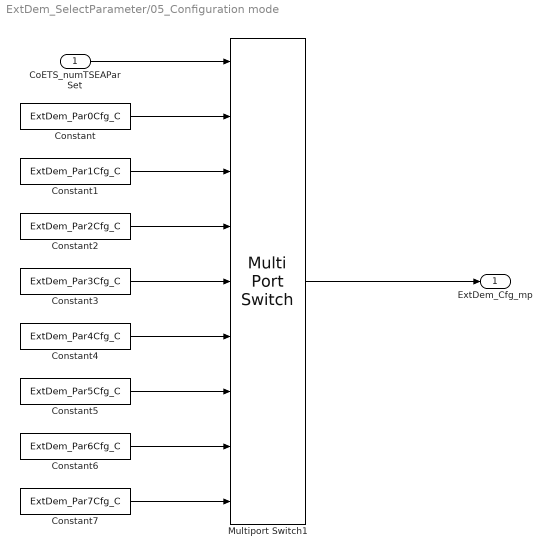
== system ExtDem_SelectParameter/05_Conﬁguration mode  ==
  CoETS_numTSEAParSet : Inport  Description=Number of requested parameter set for Engine speed governor  OutMin=0  OutMax=255  OutDataTypeStr=State_uint8
  Constant : Constant  Value=ExtDem_Par0Cfg_C
  Constant1 : Constant  Value=ExtDem_Par1Cfg_C
  Constant2 : Constant  Value=ExtDem_Par2Cfg_C
  Constant3 : Constant  Value=ExtDem_Par3Cfg_C
  Constant4 : Constant  Value=ExtDem_Par4Cfg_C
  Constant5 : Constant  Value=ExtDem_Par5Cfg_C
  Constant6 : Constant  Value=ExtDem_Par6Cfg_C
  Constant7 : Constant  Value=ExtDem_Par7Cfg_C
  Multiport Switch1 : MultiPortSwitch  DataPortOrder=Zero-based contiguous  Inputs=8
  ExtDem_Cfg_mp : Outport  Description=Configuration for EISGov structure  OutMin=0  OutMax=255  OutDataTypeStr=State_uint8
  wires:
  Multiport Switch1/1 -> ExtDem_Cfg_mp/1
  CoETS_numTSEAParSet/1 -> Multiport Switch1/1
  Constant/1 -> Multiport Switch1/2
  Constant1/1 -> Multiport Switch1/3
  Constant2/1 -> Multiport Switch1/4
  Constant3/1 -> Multiport Switch1/5
  Constant4/1 -> Multiport Switch1/6
  Constant5/1 -> Multiport Switch1/7
  Constant6/1 -> Multiport Switch1/8
  Constant7/1 -> Multiport Switch1/9

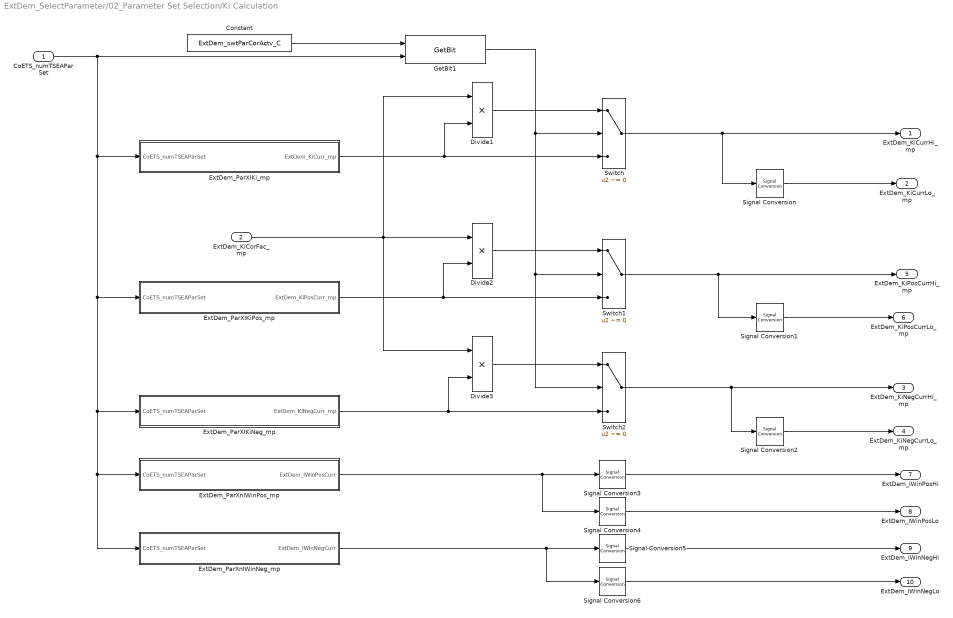
== system ExtDem_SelectParameter/02_Parameter Set Selection/Ki Calculation ==
  CoETS_numTSEAParSet : Inport  Description=Number of requested parameter set for Engine speed governor  OutMin=0  OutMax=255  OutDataTypeStr=State_uint8
  ExtDem_KiCorFac_mp : Inport  Description=Number of requested parameter set for Engine speed governor  Port=2  OutMin=-30  OutMax=30  OutDataTypeStr=Factor
  Constant : Constant  Value=ExtDem_swtParCorActv_C
  Divide1 : Product  Inputs=**  OutDataTypeStr=Inherit: Inherit via back propagation  SaturateOnIntegerOverflow=on
  Divide2 : Product  Inputs=**  OutDataTypeStr=Inherit: Inherit via back propagation  SaturateOnIntegerOverflow=on
  Divide3 : Product  Inputs=**  OutDataTypeStr=Inherit: Inherit via back propagation  SaturateOnIntegerOverflow=on
  ExtDem_ParXIKiNeg_mp : Subsystem
  ExtDem_ParXIKiPos_mp : Subsystem
  ExtDem_ParXIKi_mp : Subsystem
  ExtDem_ParXnIWinNeg_mp : Subsystem
  ExtDem_ParXnIWinPos_mp : Subsystem
  GetBit1 : CXLib/GetBit  dataTypeString=uint8  dataLength=0
      settings: AttributesFormatString=Get bit from %<dataTypeString>
  Signal Conversion{,1..6} (7 alike) : SignalConversion  OverrideOpt=off
  Switch : Switch  Criteria=u2 ~= 0
  Switch1 : Switch  Criteria=u2 ~= 0
  Switch2 : Switch  Criteria=u2 ~= 0
  ExtDem_KiCurrHi_mp : Outport  Tag=Nm/(rpm*s)  Description=Current small signal gain for the I higher component  OutMin=-18000  OutMax=18000  OutDataTypeStr=HLSDem_Ki
  ExtDem_KiCurrLo_mp : Outport  Tag=Nm/(rpm*s)  Description=Current small signal gain for the I lower component  Port=2  OutMin=-18000  OutMax=18000  OutDataTypeStr=HLSDem_Ki
  ExtDem_KiNegCurrHi_mp : Outport  Tag=Nm/(rpm*s)  Description=Current negative large signal gain for the I higher component  Port=3  OutMin=-18000  OutMax=18000  OutDataTypeStr=HLSDem_Ki
  ExtDem_KiNegCurrLo_mp : Outport  Tag=Nm/(rpm*s)  Description=Current negative large signal gain for the I lower component  Port=4  OutMin=-18000  OutMax=18000  OutDataTypeStr=HLSDem_Ki
  ExtDem_KiPosCurrHi_mp : Outport  Tag=Nm/(rpm*s)  Description=Current positive large signal gain for the I higher component  Port=5  OutMin=-18000  OutMax=18000  OutDataTypeStr=HLSDem_Ki
  ExtDem_KiPosCurrLo_mp : Outport  Tag=Nm/(rpm*s)  Description=Current positive large signal gain for the I lower component  Port=6  OutMin=-18000  OutMax=18000  OutDataTypeStr=HLSDem_Ki
  ExtDem_IWinPosHi : Outport  Tag=rpm  Description=Positive small signal window for integral higher component  Port=7  OutMin=-1000  OutMax=1000  OutDataTypeStr=EngSpeed_rpm
  ExtDem_IWinPosLo : Outport  Tag=rpm  Description=Positive small signal window for integral lower component  Port=8  OutMin=-1000  OutMax=1000  OutDataTypeStr=EngSpeed_rpm
  ExtDem_IWinNegHi : Outport  Tag=rpm  Description=Negative small signal window for integral higher component  Port=9  OutMin=-1000  OutMax=1000  OutDataTypeStr=EngSpeed_rpm
  ExtDem_IWinNegLo : Outport  Tag=rpm  Description=Negative small signal window for integral lower component  Port=10  OutMin=-1000  OutMax=1000  OutDataTypeStr=EngSpeed_rpm
  wires:
  CoETS_numTSEAParSet/1 -> GetBit1/2, ExtDem_ParXIKi_mp/1(CoETS_numTSEAParSet), ExtDem_ParXIKiPos_mp/1(CoETS_numTSEAParSet), ExtDem_ParXIKiNeg_mp/1(CoETS_numTSEAParSet), ExtDem_ParXnIWinPos_mp/1(CoETS_numTSEAParSet), ExtDem_ParXnIWinNeg_mp/1(CoETS_numTSEAParSet)
  Constant/1 -> GetBit1/1
  Divide3/1 -> Switch2/1
  Divide2/1 -> Switch1/1
  Divide1/1 -> Switch/1
  ExtDem_KiCorFac_mp/1 -> Divide3/1, Divide2/1, Divide1/1
  ExtDem_ParXIKiNeg_mp/1(ExtDem_KiNegCurr_mp) -> Switch2/3, Divide3/2
  ExtDem_ParXIKiPos_mp/1(ExtDem_KiPosCurr_mp) -> Divide2/2, Switch1/3
  ExtDem_ParXIKi_mp/1(ExtDem_KiCurr_mp) -> Divide1/2, Switch/3
  GetBit1/1 -> Switch2/2, Switch1/2, Switch/2
  Switch/1 -> ExtDem_KiCurrHi_mp/1, Signal Conversion/1
  Signal Conversion/1 -> ExtDem_KiCurrLo_mp/1
  Switch2/1 -> Signal Conversion2/1, ExtDem_KiNegCurrHi_mp/1
  Signal Conversion2/1 -> ExtDem_KiNegCurrLo_mp/1
  Switch1/1 -> Signal Conversion1/1, ExtDem_KiPosCurrHi_mp/1
  Signal Conversion1/1 -> ExtDem_KiPosCurrLo_mp/1
  ExtDem_ParXnIWinNeg_mp/1(ExtDem_IWinNegCurr) -> Signal Conversion6/1, Signal Conversion5/1
  Signal Conversion5/1 -> ExtDem_IWinNegHi/1
  Signal Conversion3/1 -> ExtDem_IWinPosHi/1
  Signal Conversion4/1 -> ExtDem_IWinPosLo/1
  Signal Conversion6/1 -> ExtDem_IWinNegLo/1
  ExtDem_ParXnIWinPos_mp/1(ExtDem_IWinPosCurr) -> Signal Conversion4/1, Signal Conversion3/1

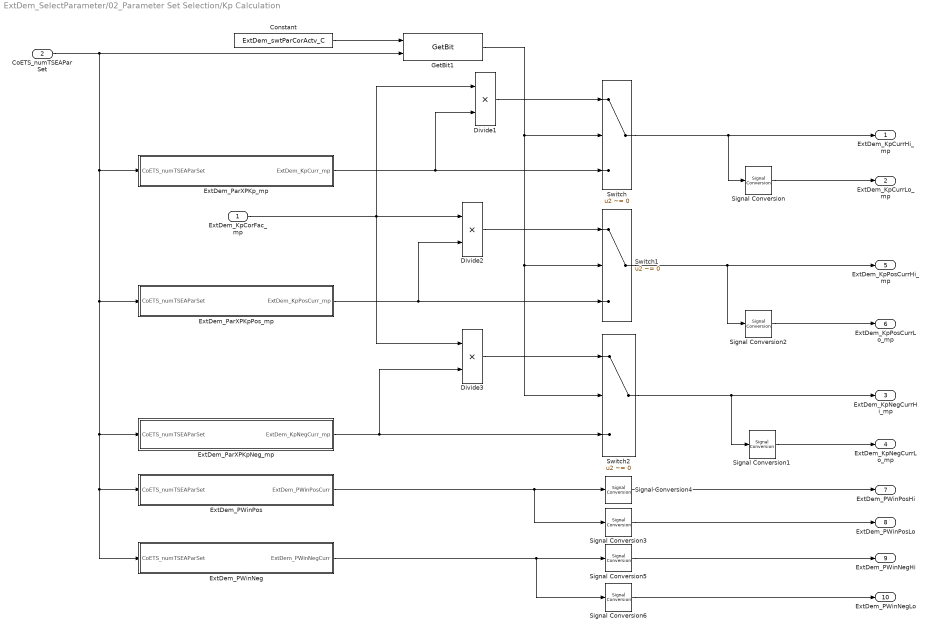
== system ExtDem_SelectParameter/02_Parameter Set Selection/Kp Calculation  ==
  ExtDem_KpCorFac_mp : Inport  Description=Number of requested parameter set for Engine speed governor  OutMin=-30  OutMax=30  OutDataTypeStr=Factor
  CoETS_numTSEAParSet : Inport  Description=Number of requested parameter set for Engine speed governor  Port=2  OutMin=0  OutMax=255  OutDataTypeStr=State_uint8
  Constant : Constant  Value=ExtDem_swtParCorActv_C
  Divide1 : Product  Inputs=**  OutDataTypeStr=Inherit: Inherit via back propagation  SaturateOnIntegerOverflow=on
  Divide2 : Product  Inputs=**  OutDataTypeStr=Inherit: Inherit via back propagation  SaturateOnIntegerOverflow=on
  Divide3 : Product  Inputs=**  OutDataTypeStr=Inherit: Inherit via back propagation  SaturateOnIntegerOverflow=on
  ExtDem_PWinNeg : Subsystem
  ExtDem_PWinPos : Subsystem
  ExtDem_ParXPKpNeg_mp : Subsystem
  ExtDem_ParXPKpPos_mp : Subsystem
  ExtDem_ParXPKp_mp : Subsystem
  GetBit1 : CXLib/GetBit  dataTypeString=uint8  dataLength=0
      settings: AttributesFormatString=Get bit from %<dataTypeString>
  Signal Conversion{,1..6} (7 alike) : SignalConversion  OverrideOpt=off
  Switch : Switch  Criteria=u2 ~= 0
  Switch1 : Switch  Criteria=u2 ~= 0
  Switch2 : Switch  Criteria=u2 ~= 0
  ExtDem_KpCurrHi_mp : Outport  Tag=Nm/rpm  Description=Current small signal gain for the P higher component  OutMin=-10000  OutMax=10000  OutDataTypeStr=HLSDem_Kp
  ExtDem_KpCurrLo_mp : Outport  Tag=Nm/rpm  Description=Current small signal gain for the P lower component  Port=2  OutMin=-10000  OutMax=10000  OutDataTypeStr=HLSDem_Kp
  ExtDem_KpNegCurrHi_mp : Outport  Tag=Nm/rpm  Description=Current negative large signal gain for the P higher component  Port=3  OutMin=-10000  OutMax=10000  OutDataTypeStr=HLSDem_Kp
  ExtDem_KpNegCurrLo_mp : Outport  Tag=Nm/rpm  Description=Current negative large signal gain for the lower P component  Port=4  OutMin=-10000  OutMax=10000  OutDataTypeStr=HLSDem_Kp
  ExtDem_KpPosCurrHi_mp : Outport  Tag=Nm/rpm  Description=Current positive large signal gain for the P higher component  Port=5  OutMin=-10000  OutMax=10000  OutDataTypeStr=HLSDem_Kp
  ExtDem_KpPosCurrLo_mp : Outport  Tag=Nm/rpm  Description=Current positive large signal gain for the P lower component  Port=6  OutMin=-10000  OutMax=10000  OutDataTypeStr=HLSDem_Kp
  ExtDem_PWinPosHi : Outport  Tag=rpm  Description=Positive small signal window for proportional higher component  Port=7  OutMin=-1000  OutMax=1000  OutDataTypeStr=EngSpeed_rpm
  ExtDem_PWinPosLo : Outport  Tag=rpm  Description=Positive small signal window for proportional lower component  Port=8  OutMin=-1000  OutMax=1000  OutDataTypeStr=EngSpeed_rpm
  ExtDem_PWinNegHi : Outport  Tag=rpm  Description=Negative small signal window for proportional higher component  Port=9  OutMin=-1000  OutMax=1000  OutDataTypeStr=EngSpeed_rpm
  ExtDem_PWinNegLo : Outport  Tag=rpm  Description=Negative small signal window for proportional lower component  Port=10  OutMin=-1000  OutMax=1000  OutDataTypeStr=EngSpeed_rpm
  wires:
  GetBit1/1 -> Switch/2, Switch2/2, Switch1/2
  ExtDem_ParXPKp_mp/1(ExtDem_KpCurr_mp) -> Divide1/2, Switch/3
  ExtDem_ParXPKpPos_mp/1(ExtDem_KpPosCurr_mp) -> Divide2/2, Switch1/3
  ExtDem_ParXPKpNeg_mp/1(ExtDem_KpNegCurr_mp) -> Switch2/3, Divide3/2
  ExtDem_KpCorFac_mp/1 -> Divide3/1, Divide2/1, Divide1/1
  Divide1/1 -> Switch/1
  Divide2/1 -> Switch1/1
  Divide3/1 -> Switch2/1
  Constant/1 -> GetBit1/1
  CoETS_numTSEAParSet/1 -> GetBit1/2, ExtDem_PWinNeg/1(CoETS_numTSEAParSet), ExtDem_PWinPos/1(CoETS_numTSEAParSet), ExtDem_ParXPKpNeg_mp/1(CoETS_numTSEAParSet), ExtDem_ParXPKpPos_mp/1(CoETS_numTSEAParSet), ExtDem_ParXPKp_mp/1(CoETS_numTSEAParSet)
  Switch/1 -> Signal Conversion/1, ExtDem_KpCurrHi_mp/1
  Signal Conversion/1 -> ExtDem_KpCurrLo_mp/1
  Switch2/1 -> ExtDem_KpNegCurrHi_mp/1, Signal Conversion1/1
  Signal Conversion1/1 -> ExtDem_KpNegCurrLo_mp/1
  Switch1/1 -> Signal Conversion2/1, ExtDem_KpPosCurrHi_mp/1
  Signal Conversion2/1 -> ExtDem_KpPosCurrLo_mp/1
  ExtDem_PWinPos/1(ExtDem_PWinPosCurr) -> Signal Conversion3/1, Signal Conversion4/1
  ExtDem_PWinNeg/1(ExtDem_PWinNegCurr) -> Signal Conversion6/1, Signal Conversion5/1
  Signal Conversion4/1 -> ExtDem_PWinPosHi/1
  Signal Conversion5/1 -> ExtDem_PWinNegHi/1
  Signal Conversion3/1 -> ExtDem_PWinPosLo/1
  Signal Conversion6/1 -> ExtDem_PWinNegLo/1

== system ExtDem_SelectParameter/03_Feedback Factor / inner feedback factors  ==
  CoETS_numTSEAParSet : Inport  Description=Number of requested parameter set for Engine speed governor  OutMin=0  OutMax=255  OutDataTypeStr=State_uint8
  InrtVehCurr : Subsystem
  facFdbkTrqLosHi : Subsystem
  facFdbkTrqLosLo : Subsystem
  tiFltTrqLosEstCurr : Subsystem
  ExtDem_facFdbkTrqLosHi : Outport  Tag=rpm/Nm  Description=inner feedback factor for the upper setpoint  OutMin=-20  OutMax=20  OutDataTypeStr=FdbkNm2rpm_rpm_Nm
  ExtDem_facFdbkTrqLosLo : Outport  Tag=rpm/Nm  Description=inner feedback factor for the lower setpoint  Port=2  OutMin=-20  OutMax=20  OutDataTypeStr=FdbkNm2rpm_rpm_Nm
  ExtDem_InrtVehCurr : Outport  Tag=Nm/(rpm/s)  Description=Mass inirtia for EISGov torque loss estimation  Port=3  OutMin=-50  OutMax=50  OutDataTypeStr=HLSDem_Inrt
  ExtDem_tiFltTrqLosEstCurr : Outport  Tag=s  Description=Time constant for EISGov torque loss calculation  Port=4  OutMin=-180  OutMax=180  OutDataTypeStr=Time_s
  wires:
  facFdbkTrqLosLo/1(ExtDem_facFdbkTrqLosLo) -> ExtDem_facFdbkTrqLosLo/1
  CoETS_numTSEAParSet/1 -> tiFltTrqLosEstCurr/1(CoETS_numTSEAParSet), InrtVehCurr/1(CoETS_numTSEAParSet), facFdbkTrqLosLo/1(CoETS_numTSEAParSet), facFdbkTrqLosHi/1(CoETS_numTSEAParSet)
  facFdbkTrqLosHi/1(ExtDem_facFdbkTrqLosHi) -> ExtDem_facFdbkTrqLosHi/1
  InrtVehCurr/1(ExtDem_InrtVehCurr) -> ExtDem_InrtVehCurr/1
  tiFltTrqLosEstCurr/1(ExtDem_tiFltTrqLosEstCurr) -> ExtDem_tiFltTrqLosEstCurr/1
